simulink model "KonNarxModel1"  (R2017a)
settings: Solver=VariableStepAuto  StartTime=0.0  StopTime=500  RelTol=1e-3
settings Model: Creator=Korisnik  LastModifiedBy=Korisnik

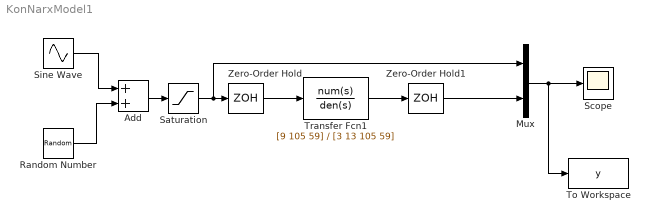
== system KonNarxModel1 ==
  Add : Sum
  Mux : Mux  Inputs=2
  Random Number : RandomNumber  Variance=0.1  SampleTime=0.1
  Saturation : Saturate  UpperLimit=5  LowerLimit=-5
  Scope : Scope
  Sine Wave : Sin  Amplitude=4  Frequency=0.025  SampleTime=0.1
  To Workspace : ToWorkspace  VariableName=y  SampleTime=-1
  Transfer Fcn1 : TransferFcn  Numerator=[9 105 59]  Denominator=[3 13 105 59]
  Zero-Order Hold : ZeroOrderHold  SampleTime=0.1
  Zero-Order Hold1 : ZeroOrderHold  SampleTime=0.1
  wires:
  Zero-Order Hold/1 -> Transfer Fcn1/1
  Mux/1 -> To Workspace/1, Scope/1
  Random Number/1 -> Add/2
  Sine Wave/1 -> Add/1
  Zero-Order Hold1/1 -> Mux/2
  Add/1 -> Saturation/1
  Transfer Fcn1/1 -> Zero-Order Hold1/1
  Saturation/1 -> Mux/1, Zero-Order Hold/1
